simulink model "Ass3Q2_3"  (R2018b)
settings: Solver=VariableStepAuto  StartTime=0.0  StopTime=40  RelTol=1e-3
values from neighbouring files (symbols this model uses):
  D = [X(3),0,c_0]    [Adaptive3.m]
undefined symbols (not defined in the file or in its folder): ss_mo, ss_pl, sys_m
settings Model: Creator=bigfoot  LastModifiedBy=bigfoot

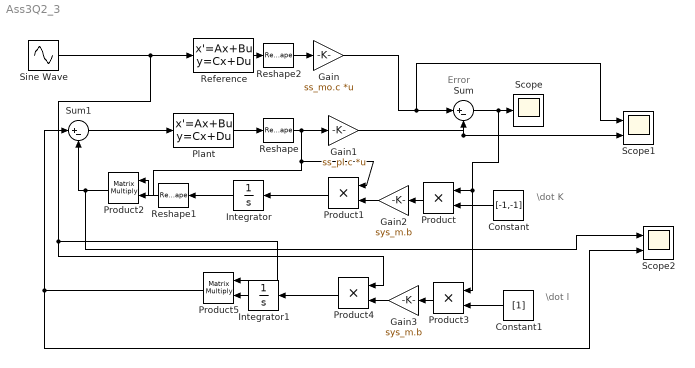
== system Ass3Q2_3 ==
  note: \dot l
  note: \dot K
  note: Error
  Constant : Constant  Value=[-1,-1]
  Constant1 : Constant  Value=[1]
  Gain : Gain  Gain=ss_mo.c  Multiplication=Matrix(K*u)
  Gain1 : Gain  Gain=ss_pl.c  Multiplication=Matrix(K*u)
  Gain2 : Gain  Gain=sys_m.b
  Gain3 : Gain  Gain=sys_m.b
  Integrator : Integrator
  Integrator1 : Integrator
  Plant : StateSpace  A=ss_pl.a  B=ss_pl.b  C=eye(2)  D=[0;0]  InitialCondition=[0.4,0.2]
  Product{,1,3..4} (4 alike) : Product
  Product2 : Product  Multiplication=Matrix(*)
  Product5 : Product  Multiplication=Matrix(*)
  Reference : StateSpace  A=ss_mo.a  B=ss_mo.b  C=eye(2)  D=[0;0]  InitialCondition=0
  Reshape : Reshape  OutputDimensionality=Column vector (2-D)
  Reshape1 : Reshape  OutputDimensionality=Row vector (2-D)
  Reshape2 : Reshape  OutputDimensionality=Column vector (2-D)
  Scope : Scope
  Scope1 : Scope  NumInputPorts=2
  Scope2 : Scope  NumInputPorts=2
  Sine Wave : Sin  SampleTime=0
  Sum : Sum  Inputs=|+-
  Sum1 : Sum  Inputs=|+-
  wires:
  Sum/1 -> Product3/1, Product/1, Scope/1
  Gain/1 -> Scope1/1, Sum/1
  Gain1/1 -> Scope1/2, Sum/2
  Constant/1 -> Product/2
  Product/1 -> Gain2/1
  Gain2/1 -> Product1/2
  Product1/1 -> Integrator/1
  Plant/1 -> Reshape/1
  Integrator/1 -> Reshape1/1
  Reshape/1 -> Gain1/1, Product2/2, Product1/1
  Reshape1/1 -> Product2/1
  Gain3/1 -> Product4/2
  Product3/1 -> Gain3/1
  Constant1/1 -> Product3/2
  Product4/1 -> Integrator1/1
  Integrator1/1 -> Product5/2
  Sine Wave/1 -> Product5/1, Product4/1, Reference/1
  Sum1/1 -> Plant/1
  Product2/1 -> Scope2/1, Sum1/2
  Product5/1 -> Sum1/1, Scope2/2
  Reference/1 -> Reshape2/1
  Reshape2/1 -> Gain/1
